simulink model "cblocks"  (Simulink 2.20)
settings: Solver=ode45  StartTime=0.0  StopTime=999999  MaxStep=10  RelTol=1e-3  AbsTol=1e-3
undefined symbols (not defined in the file or in its folder): TSAMPLE
settings Model: SaveTime=off  SaveOutput=off  ConsistencyChecking=off  RTWPlaceOutputsASAP=off

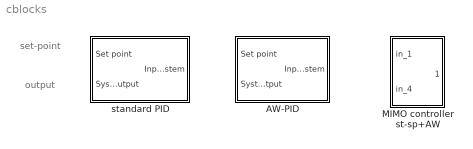
== system cblocks ==
  note: set-point
  note: output
  "AW-PID " : Subsystem  mask(Anti-windup PID ){@1=[.05, 3, 0.5], @2=1/60, @3=0.1, @4=1/60, @5=[0.7 -0.3]}
      mask prompts: @1 "Gain kp - Integral time ki - Derivative time kd"; @2 "Pseudo-derivative filter time constant"; @3 "Error lowpass filter Time constant"; @4 "Sampling Time"; @5 "Saturation Limits [umax umin]"
      mask help: Discrete PID with Anti-windup and with lowpass filter
      mask init:
      | kp=@1(1);ki=@1(2);kd=@1(3);SAM=@2;TF=@3;DT=@4;umax=@5(1);umin=@5(2);
      mask Display: disp('AW-PID+filter')
  MIMO controller st-sp+AW : Subsystem
  standard PID : Subsystem  mask(Discrete PID ){@1=[.05, 3, 0.5], @2=1/60, @3=0.1, @4=1/60}
      mask prompts: @1 "Gain kp - Integral time ki - Derivative time kd"; @2 "Pseudo-derivative filter time constant"; @3 "Error lowpass filter Time constant"; @4 "Sampling Time"
      mask help: Discrete PID with lowpass filter
      mask init:
      | kp=@1(1);ki=@1(2);kd=@1(3);SAM=@2;TF=@3;DT=@4;
      mask Display: disp('PID+filter')

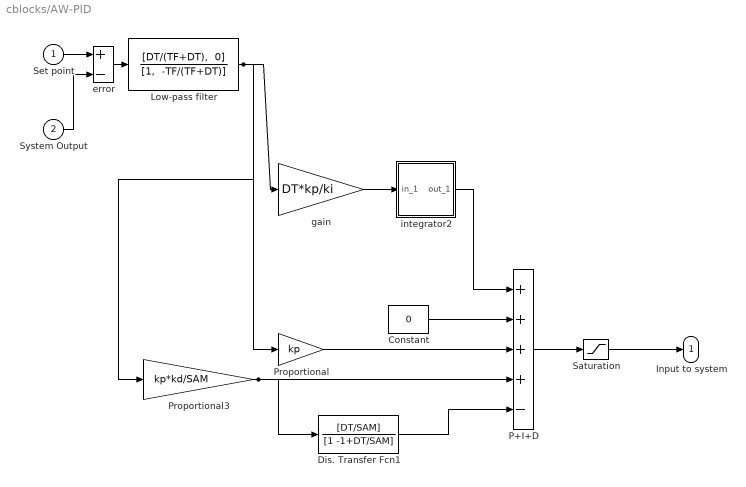
== system cblocks/AW-PID  ==
  Set point : Inport  Port=1  PortWidth=-1  SampleTime=-1
  System Output : Inport  Port=2  PortWidth=-1  SampleTime=-1
  Constant : Constant  Value=0
  Dis. Transfer Fcn1 : DiscreteTransferFcn  Numerator=[DT/SAM]  Denominator=[1 -1+DT/SAM]  SampleTime=DT
  Low-pass filter : DiscreteTransferFcn  Numerator="[DT/(TF+DT),  0]"  Denominator="[1,  -TF/(TF+DT)]"  SampleTime=DT
  P+I+D : Sum  Inputs=++++-
  Proportional : Gain  Gain=kp
  Proportional3 : Gain  Gain=kp*kd/SAM
  Saturation : Saturate  UpperLimit=umax  LowerLimit=umin
  error : Sum  Inputs=+-
  gain : Gain  Gain=DT*kp/ki
  integrator2 : Subsystem  mask(Anti windup intgrator){@1=umax, @2=umin, @3=DT}
      mask prompts: @1 "umax"; @2 "umin"; @3 "sampling time"
      mask help: Integral with anti-windup
      mask init:
      | umax=@1 ; umin =@2 ;DT=@3;
      mask Display: disp('DT-I-AW')
  Input to system : Outport  Port=1  InitialOutput=0
  wires:
  Constant/1 -> P+I+D/2
  Saturation/1 -> Input to system/1
  P+I+D/1 -> Saturation/1
  gain/1 -> integrator2/1(in_1)
  Proportional/1 -> P+I+D/3
  Dis. Transfer Fcn1/1 -> P+I+D/5
  Low-pass filter/1 -> gain/1, Proportional3/1, Proportional/1
  Proportional3/1 -> P+I+D/4, Dis. Transfer Fcn1/1
  System Output/1 -> error/2
  Set point/1 -> error/1
  error/1 -> Low-pass filter/1
  integrator2/1(out_1) -> P+I+D/1

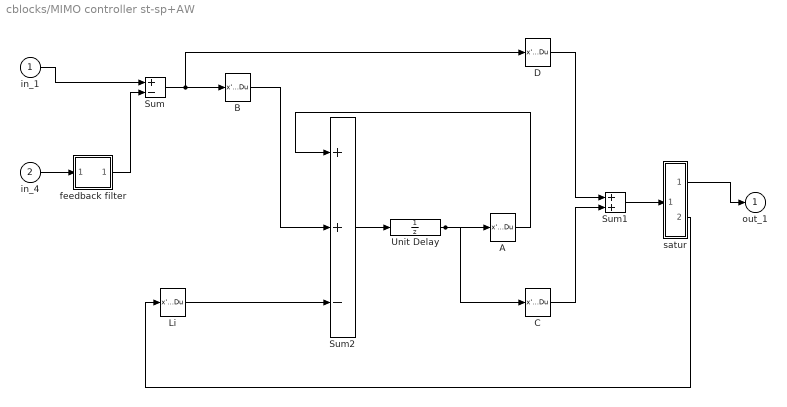
== system cblocks/MIMO controller st-sp+AW ==
  in_1 : Inport  Port=1  PortWidth=-1  SampleTime=-1
  in_4 : Inport  Port=2  PortWidth=-1  SampleTime=-1
  A : StateSpace  A=[]  B=[]  C=[]  D=K  X0=0  mask(Matrix Gain){@1=Aci}
      mask prompts: @1 "Gain matrix:"
      mask help: Matrix Gain.
      mask init:
      | K = @1;
      mask Help: Multiplies input vector by entered matrix to produce output vector (y=Au).
      mask Display: disp('K')
  B : StateSpace  A=[]  B=[]  C=[]  D=K  X0=0  mask(Matrix Gain){@1=Bci}
      mask prompts: @1 "Gain matrix:"
      mask help: Matrix Gain.
      mask init:
      | K = @1;
      mask Help: Multiplies input vector by entered matrix to produce output vector (y=Au).
      mask Display: disp('K')
  C : StateSpace  A=[]  B=[]  C=[]  D=K  X0=0  mask(Matrix Gain){@1=Cci}
      mask prompts: @1 "Gain matrix:"
      mask help: Matrix Gain.
      mask init:
      | K = @1;
      mask Help: Multiplies input vector by entered matrix to produce output vector (y=Au).
      mask Display: disp('K')
  D : StateSpace  A=[]  B=[]  C=[]  D=K  X0=0  mask(Matrix Gain){@1=Dci}
      mask prompts: @1 "Gain matrix:"
      mask help: Matrix Gain.
      mask init:
      | K = @1;
      mask Help: Multiplies input vector by entered matrix to produce output vector (y=Au).
      mask Display: disp('K')
  Li : StateSpace  A=[]  B=[]  C=[]  D=K  X0=0  mask(Matrix Gain){@1=LDi}
      mask prompts: @1 "Gain matrix:"
      mask help: Matrix Gain.
      mask init:
      | K = @1;
      mask Help: Multiplies input vector by entered matrix to produce output vector (y=Au).
      mask Display: disp('K')
  Sum : Sum  Inputs=+-
  Sum1 : Sum  Inputs=++
  Sum2 : Sum  Inputs=++-
  Unit Delay : UnitDelay  X0=0  SampleTime=TSAMPLE
  feedback filter : Subsystem
  satur : Subsystem  mask(saturations and dead zones){@1=[1 1 1], @2=[0 0 0]}
      mask prompts: @1 "max 1-2-3"; @2 "min 1-2-3"
      mask help: sats+dzn
      mask init:
      | Upmax=@1;Upmin=@2;
  out_1 : Outport  Port=1  InitialOutput=0
  wires:
  in_1/1 -> Sum/1
  Sum/1 -> B/1, D/1
  D/1 -> Sum1/1
  Sum2/1 -> Unit Delay/1
  A/1 -> Sum2/1
  B/1 -> Sum2/2
  C/1 -> Sum1/2
  Unit Delay/1 -> A/1, C/1
  Li/1 -> Sum2/3
  Sum1/1 -> satur/1(in_1)
  satur/1(out_1) -> out_1/1
  satur/2(out_2) -> Li/1
  in_4/1 -> feedback filter/1(in_1)
  feedback filter/1(out_1) -> Sum/2

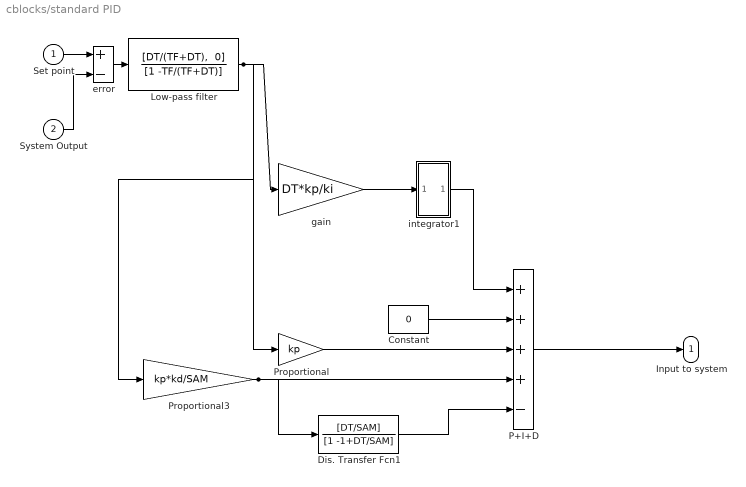
== system cblocks/standard PID ==
  Set point : Inport  Port=1  PortWidth=-1  SampleTime=-1
  System Output : Inport  Port=2  PortWidth=-1  SampleTime=-1
  Constant : Constant  Value=0
  Dis. Transfer Fcn1 : DiscreteTransferFcn  Numerator=[DT/SAM]  Denominator=[1 -1+DT/SAM]  SampleTime=DT
  Low-pass filter : DiscreteTransferFcn  Numerator="[DT/(TF+DT),  0]"  Denominator=[1 -TF/(TF+DT)]  SampleTime=DT
  P+I+D : Sum  Inputs=++++-
  Proportional : Gain  Gain=kp
  Proportional3 : Gain  Gain=kp*kd/SAM
  error : Sum  Inputs=+-
  gain : Gain  Gain=DT*kp/ki
  integrator1 : Subsystem
  Input to system : Outport  Port=1  InitialOutput=0
  wires:
  Constant/1 -> P+I+D/2
  gain/1 -> integrator1/1(in_1)
  Proportional/1 -> P+I+D/3
  Dis. Transfer Fcn1/1 -> P+I+D/5
  Low-pass filter/1 -> gain/1, Proportional3/1, Proportional/1
  Proportional3/1 -> P+I+D/4, Dis. Transfer Fcn1/1
  System Output/1 -> error/2
  Set point/1 -> error/1
  error/1 -> Low-pass filter/1
  integrator1/1(out_1) -> P+I+D/1
  P+I+D/1 -> Input to system/1

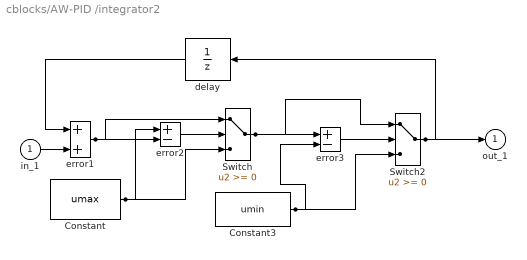
== system cblocks/AW-PID /integrator2 ==
  in_1 : Inport  Port=1  PortWidth=-1  SampleTime=-1
  Constant : Constant  Value=umax
  Constant3 : Constant  Value=umin
  Switch : Switch  Threshold=0
  Switch2 : Switch  Threshold=0
  delay : DiscreteTransferFcn  Orientation=left  Numerator=[1]  Denominator=[1 0]  SampleTime=DT
  error1 : Sum  Inputs=++
  error2 : Sum  Inputs=+-
  error3 : Sum  Inputs=+-
  out_1 : Outport  Port=1  InitialOutput=0
  wires:
  in_1/1 -> error1/2
  Switch2/1 -> out_1/1, delay/1
  Switch/1 -> Switch2/1, error3/1
  Constant3/1 -> Switch2/3, error3/2
  error3/1 -> Switch2/2
  error1/1 -> Switch/1, error2/2
  Constant/1 -> Switch/3, error2/1
  error2/1 -> Switch/2
  delay/1 -> error1/1

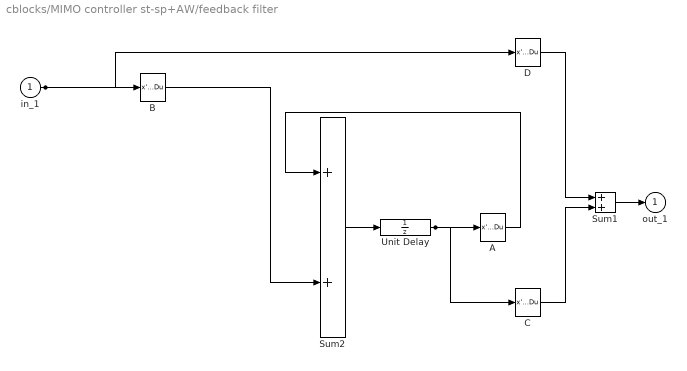
== system cblocks/MIMO controller st-sp+AW/feedback filter ==
  in_1 : Inport  Port=1  PortWidth=-1  SampleTime=-1
  A : StateSpace  A=[]  B=[]  C=[]  D=K  X0=0  mask(Matrix Gain){@1=Afo}
      mask prompts: @1 "Gain matrix:"
      mask help: Matrix Gain.
      mask init:
      | K = @1;
      mask Help: Multiplies input vector by entered matrix to produce output vector (y=Au).
      mask Display: disp('K')
  B : StateSpace  A=[]  B=[]  C=[]  D=K  X0=0  mask(Matrix Gain){@1=Bfo}
      mask prompts: @1 "Gain matrix:"
      mask help: Matrix Gain.
      mask init:
      | K = @1;
      mask Help: Multiplies input vector by entered matrix to produce output vector (y=Au).
      mask Display: disp('K')
  C : StateSpace  A=[]  B=[]  C=[]  D=K  X0=0  mask(Matrix Gain){@1=Cfo}
      mask prompts: @1 "Gain matrix:"
      mask help: Matrix Gain.
      mask init:
      | K = @1;
      mask Help: Multiplies input vector by entered matrix to produce output vector (y=Au).
      mask Display: disp('K')
  D : StateSpace  A=[]  B=[]  C=[]  D=K  X0=0  mask(Matrix Gain){@1=Dfo}
      mask prompts: @1 "Gain matrix:"
      mask help: Matrix Gain.
      mask init:
      | K = @1;
      mask Help: Multiplies input vector by entered matrix to produce output vector (y=Au).
      mask Display: disp('K')
  Sum1 : Sum  Inputs=++
  Sum2 : Sum  Inputs=++
  Unit Delay : UnitDelay  X0=0  SampleTime=TSAMPLE
  out_1 : Outport  Port=1  InitialOutput=0
  wires:
  Unit Delay/1 -> C/1, A/1
  C/1 -> Sum1/2
  B/1 -> Sum2/2
  A/1 -> Sum2/1
  Sum2/1 -> Unit Delay/1
  Sum1/1 -> out_1/1
  D/1 -> Sum1/1
  in_1/1 -> D/1, B/1

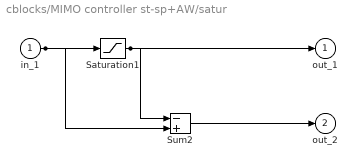
== system cblocks/MIMO controller st-sp+AW/satur ==
  in_1 : Inport  Port=1  PortWidth=-1  SampleTime=-1
  Saturation1 : Saturate  UpperLimit=Upmax  LowerLimit=Upmin
  Sum2 : Sum  Inputs=-+
  out_1 : Outport  Port=1  InitialOutput=0
  out_2 : Outport  Port=2  InitialOutput=0
  wires:
  Saturation1/1 -> out_1/1, Sum2/1
  Sum2/1 -> out_2/1
  in_1/1 -> Sum2/2, Saturation1/1

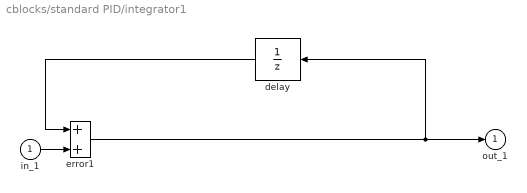
== system cblocks/standard PID/integrator1 ==
  in_1 : Inport  Port=1  PortWidth=-1  SampleTime=-1
  delay : DiscreteTransferFcn  Orientation=left  Numerator=[1]  Denominator=[1 0]  SampleTime=DT
  error1 : Sum  Inputs=++
  out_1 : Outport  Port=1  InitialOutput=0
  wires:
  in_1/1 -> error1/2
  error1/1 -> out_1/1, delay/1
  delay/1 -> error1/1
